simulink model "SimulinkAnalysisofCheetahTail"  (R2022a)
settings: Solver=ode4  StartTime=0.0  StopTime=1.5  FixedStep=0.001  RelTol=1e-3
undefined symbols (not defined in the file): B_cg_H, B_con_H, B_con_L, bar_len, cd_table, Cf, cl_table, g, gear_ratio, int_point_bar, int_point_tail, ITail, M_add, M_cg_H, M_cg_L, M_cg_W, Mb, Mm, Mt, psi3, rho, T_cg_H, T_fur_gap, T_length, T_width_major, T_width_minor, th2_initial, torque_constant, uncertainty_Forces, uncertainty_Position, Vf, windspeed
(part 18 of 21)

== matlab function SimulinkAnalysisofCheetahTail/Model/Forces/CD_CL_tail_3/aoa_tail_3 ==
  data: int_point_tail input; q input; dq input; aoa_tail_3 output; psi3 parameter; windspeed parameter; B_con_H parameter; B_con_L parameter; M_cg_H parameter; M_cg_L parameter; M_cg_W parameter; T_fur_gap parameter; T_length parameter; bar_len parameter
function aoa_tail_3  = aoa_tail_3( int_point_tail,q,dq, psi3, windspeed, B_con_H, B_con_L, M_cg_H, M_cg_L, M_cg_W, T_fur_gap, T_length, bar_len)
%#codegen
[x,y,z,phi1,th1,psi1,phi2,th2] = deal(q(1),q(2),q(3),q(4),q(5),q(6),q(7),q(8));
[dx,dy,dz,dphi1,dth1,dpsi1,dphi2,dth2] = deal(dq(1),dq(2),dq(3),dq(4),dq(5),dq(6),dq(7),dq(8));
%    This function was generated by the Symbolic Math Toolbox version 9.0.
%    09-Feb-2022 11:07:29

t2 = cos(phi1);
t3 = cos(phi2);
t4 = cos(psi1);
t5 = cos(psi3);
t6 = cos(th1);
t7 = cos(th2);
t8 = sin(phi1);
t9 = sin(phi2);
t10 = sin(psi1);
t11 = sin(psi3);
t12 = sin(th1);
t13 = sin(th2);
t14 = M_cg_L+x;
t15 = M_cg_W+y;
t16 = M_cg_H+z;
t24 = T_length./2.0;
t25 = bar_len./2.0;
t26 = int_point_tail./2.0;
t17 = B_con_L.*t6;
t18 = B_con_L.*t12;
t19 = t2.*t4;
t20 = t2.*t10;
t21 = t4.*t8;
t22 = t7.*t12;
t23 = t8.*t10;
t27 = B_con_H.*t2.*t6;
t29 = t6.*t14;
t30 = B_con_H.*t2.*t12;
t31 = B_con_H.*t6.*t8;
t34 = t12.*t14;
t36 = -t26;
t37 = t3.*t12.*t13;
t38 = t8.*t9.*t12;
t40 = t9.*t12.*t13;
t41 = t4.*t6.*t7;
t42 = t2.*t6.*t9;
t43 = t3.*t6.*t8;
t45 = t2.*t6.*t13;
t46 = t3.*t6.*t13;
t48 = t6.*t7.*t10;
t49 = t6.*t8.*t9;
t54 = t2.*t6.*t15;
t56 = t2.*t6.*t16;
t59 = t6.*t8.*t15;
t60 = t2.*t12.*t16;
t61 = t6.*t8.*t16;
t63 = t8.*t12.*t15;
t69 = t2.*t3.*t6.*t7;
t80 = t4.*t6.*t9.*t13;
t83 = t6.*t9.*t10.*t13;
t28 = t4.*t17;
t32 = t4.*t18;
t33 = t10.*t17;
t35 = t10.*t18;
t39 = t12.*t23;
t44 = t12.*t19;
t47 = t3.*t22;
t50 = t12.*t20;
t51 = t12.*t21;
t52 = B_con_H.*t6.*t19;
t53 = t4.*t29;
t55 = B_con_H.*t6.*t20;
t57 = t4.*t34;
t58 = t10.*t29;
t62 = t10.*t34;
t64 = -t30;
t65 = -t31;
t66 = -t38;
t68 = -t40;
t70 = t3.*t41;
t71 = t3.*t45;
t73 = t7.*t42;
t74 = t7.*t43;
t75 = t4.*t46;
t76 = t3.*t48;
t77 = t6.*t9.*t21;
t78 = t4.*t37;
t79 = t10.*t46;
t81 = t6.*t9.*t23;
t82 = t10.*t37;
t85 = -t48;
t86 = t6.*t16.*t19;
t87 = t6.*t15.*t21;
t88 = t6.*t16.*t20;
t89 = t6.*t15.*t23;
t90 = -t54;
t91 = -t59;
t92 = -t60;
t93 = -t61;
t94 = t3.*t6.*t7.*t19;
t95 = t3.*t6.*t7.*t20;
t96 = -t69;
t101 = t22+t45;
t120 = t24+t25+t36;
t67 = -t39;
t72 = t2.*t47;
t84 = -t44;
t97 = -t75;
t98 = -t76;
t99 = -t87;
t100 = -t89;
t102 = t20+t51;
t103 = t21+t50;
t104 = -t94;
t105 = -t95;
t111 = t11.*t101;
t115 = t42+t74;
t119 = t47+t71;
t155 = t37+t49+t96;
t157 = t43+t68+t73;
t106 = B_con_H.*t102;
t107 = B_con_H.*t103;
t108 = t19+t67;
t109 = t23+t84;
t110 = t3.*t102;
t112 = t9.*t102;
t113 = t9.*t103;
t114 = t13.*t103;
t121 = t15.*t102;
t122 = t15.*t103;
t123 = t16.*t102;
t124 = t16.*t103;
t126 = t3.*t7.*t103;
t130 = -t111;
t134 = T_fur_gap.*t115;
t135 = T_fur_gap.*t119;
t136 = int_point_tail.*t115;
t137 = int_point_tail.*t119;
t156 = t46+t66+t72;
t159 = T_fur_gap.*t155;
t161 = T_fur_gap.*t157;
t162 = int_point_tail.*t155;
t164 = int_point_tail.*t157;
t167 = t5.*t157;
t174 = t77+t78+t104;
t175 = t81+t82+t105;
t180 = t115.*t120;
t181 = t119.*t120;
t188 = t120.*t155;
t190 = t120.*t157;
t116 = B_con_H.*t108;
t117 = B_con_H.*t109;
t118 = -t107;
t125 = t7.*t110;
t127 = t3.*t114;
t128 = t7.*t113;
t129 = t3.*t108;
t131 = t9.*t108;
t132 = t9.*t109;
t133 = t13.*t109;
t138 = t15.*t108;
t139 = t15.*t109;
t140 = -t122;
t141 = t16.*t108;
t142 = t16.*t109;
t143 = -t124;
t145 = t3.*t7.*t109;
t154 = t85+t114;
t160 = T_fur_gap.*t156;
t163 = int_point_tail.*t156;
t166 = -t11.*(t48-t114);
t176 = T_fur_gap.*t174;
t177 = int_point_tail.*t174;
t178 = T_fur_gap.*t175;
t179 = int_point_tail.*t175;
t189 = t120.*t156;
t195 = t130+t167;
t206 = t120.*t174;
t207 = t120.*t175;
t220 = t135+t137+t181;
t223 = t161+t164+t190;
t224 = t65+t90+t93+t134+t136+t180;
t227 = t18+t27+t34+t56+t91+t159+t162+t188;
t144 = t7.*t129;
t146 = -t125;
t147 = t3.*t133;
t148 = t7.*t132;
t149 = -t129;
t150 = -t138;
t151 = -t139;
t158 = t41+t133;
t169 = t98+t127;
t171 = -T_fur_gap.*(t76-t127);
t173 = -int_point_tail.*(t76-t127);
t185 = -T_fur_gap.*(t125-t132);
t187 = -int_point_tail.*(t125-t132);
t191 = t79+t126+t131;
t194 = t97+t112+t145;
t199 = -t120.*(t76-t127);
t214 = -t120.*(t125-t132);
t228 = t17+t29+t63+t64+t92+t160+t163+t189;
t229 = t35+t55+t62+t88+t100+t178+t179+t207;
t230 = t32+t52+t57+t86+t99+t176+t177+t206;
t152 = -t144;
t153 = -t148;
t165 = t11.*t158;
t168 = t70+t147;
t183 = t132+t146;
t192 = T_fur_gap.*t191;
t193 = int_point_tail.*t191;
t197 = t83+t128+t149;
t200 = T_fur_gap.*t194;
t202 = int_point_tail.*t194;
t215 = t120.*t191;
t216 = t120.*t194;
t226 = t171+t173+t199;
t233 = t106+t123+t151+t185+t187+t214;
t170 = T_fur_gap.*t168;
t172 = int_point_tail.*t168;
t182 = t113+t152;
t196 = t80+t110+t153;
t198 = t120.*t168;
t203 = T_fur_gap.*t197;
t205 = int_point_tail.*t197;
t209 = t5.*t197;
t210 = -t200;
t211 = -t202;
t218 = t120.*t197;
t219 = -t216;
t235 = t33+t58+t118+t143+t150+t192+t193+t215;
t184 = T_fur_gap.*t182;
t186 = int_point_tail.*t182;
t201 = T_fur_gap.*t196;
t204 = int_point_tail.*t196;
t208 = t5.*t196;
t212 = -t209;
t213 = t120.*t182;
t217 = t120.*t196;
t225 = t170+t172+t198;
t232 = t203+t205+t218;
t236 = t28+t53+t117+t121+t142+t210+t211+t219;
t221 = t165+t208;
t222 = t166+t212;
t231 = t201+t204+t217;
t234 = t116+t140+t141+t184+t186+t213;
et1 = dphi1.*(t234.*(t209+t11.*(t48-t114))+(t111-t167).*(t31+t54+t61-t134-t136-t180)+t221.*(-t106-t123+t139+T_fur_gap.*(t125-t132)+int_point_tail.*(t125-t132)+t120.*(t125-t132))-t227.*(t5.*(t7.*t49-t2.*t3.*t6)-t6.*t8.*t11.*t13)+t236.*(t5.*(t3.*t109+t7.*t112)-t11.*t13.*t102)-t235.*(t5.*(t3.*t103+t7.*t131)-t11.*t13.*t108))+dphi2.*(t232.*(t209+t11.*(t48-t114))+t221.*t231-t223.*(t111-t167)-t5.*t155.*t227-t5.*t191.*t235+t5.*t194.*t236);
et2 = dth1.*(t229.*(t209+t11.*(t48-t114))+t221.*t230-t228.*(t111-t167)-t227.*(t11.*(t6.*t7-t2.*t12.*t13)+t5.*(t3.*t8.*t12+t6.*t9.*t13+t2.*t9.*t22))+t236.*(t11.*(t4.*t22+t6.*t13.*t19)-t5.*(t4.*t68+t3.*t6.*t21+t6.*t7.*t9.*t19))+t235.*(t11.*(t10.*t22+t6.*t13.*t20)-t5.*(t10.*t68+t3.*t6.*t23+t6.*t7.*t9.*t20)))+dy.*(t108.*(t209+t11.*(t48-t114))-t102.*t221+t6.*t8.*(t111-t167))-dz.*(-t103.*(t209+t11.*(t48-t114))+t109.*t221+t2.*t6.*(t111-t167));
et3 = -dth2.*(-t227.*(t11.*(t12.*t13-t2.*t6.*t7)-t5.*(t9.*t22+t13.*t42))-t235.*(t11.*(t7.*t103+t6.*t10.*t13)-t5.*(t9.*t48-t13.*t113))+t236.*(t11.*(t7.*t109-t4.*t6.*t13)+t5.*(t9.*t41+t13.*t132))+t221.*t225+(t209+t11.*(t48-t114)).*(T_fur_gap.*(t76-t127)+int_point_tail.*(t76-t127)+t120.*(t76-t127))+t220.*(t111-t167))-dx.*(t12.*(t111-t167)+t6.*t10.*(t209+t11.*(t48-t114))+t4.*t6.*t221)+t5.*windspeed.*(t209+t11.*(t48-t114))+t11.*t221.*windspeed;
et4 = -dphi1.*(t155.*(t31+t54+t61-t134-t136-t180)-t115.*t227+t182.*t235+t191.*t234+t236.*(t125-t132)-t194.*(-t106-t123+t139+T_fur_gap.*(t125-t132)+int_point_tail.*(t125-t132)+t120.*(t125-t132)))+dth2.*(t119.*t227+t155.*t220+t168.*t236-t194.*t225+t191.*(T_fur_gap.*(t76-t127)+int_point_tail.*(t76-t127)+t120.*(t76-t127))+t235.*(t76-t127))-dy.*(t102.*t194+t108.*t191+t6.*t8.*t155)-dz.*(t103.*t191+t109.*t194-t2.*t6.*t155)+dphi2.*(t155.*t223+t157.*t227-t191.*t232+t194.*t231-t196.*t236-t197.*t235);
et5 = dth1.*(t155.*t228+t156.*t227-t174.*t236-t175.*t235-t191.*t229+t194.*t230)+dx.*(t12.*t155-t4.*t6.*t194+t6.*t10.*t191)-t5.*t191.*windspeed+t11.*t194.*windspeed;
aoa_tail_3 = th2-atan((et4+et5)./(et1+et2+et3));

== matlab function SimulinkAnalysisofCheetahTail/Model/Forces/CD_CL_tail_4/v_tail_4 ==
  data: int_point_tail input; q input; dq input; v_tail_4_speed output; psi3 parameter; windspeed parameter; B_con_H parameter; B_con_L parameter; M_cg_H parameter; M_cg_L parameter; M_cg_W parameter; T_fur_gap parameter; T_length parameter; bar_len parameter
function v_tail_4_speed = v_tail_4(int_point_tail,q,dq, psi3, windspeed, B_con_H, B_con_L, M_cg_H, M_cg_L, M_cg_W, T_fur_gap, T_length, bar_len)
%#codegen
[x,y,z,phi1,th1,psi1,phi2,th2] = deal(q(1),q(2),q(3),q(4),q(5),q(6),q(7),q(8));
[dx,dy,dz,dphi1,dth1,dpsi1,dphi2,dth2] = deal(dq(1),dq(2),dq(3),dq(4),dq(5),dq(6),dq(7),dq(8));
%    This function was generated by the Symbolic Math Toolbox version 9.0.
%    09-Feb-2022 11:07:32

t2 = cos(phi1);
t3 = cos(phi2);
t4 = cos(psi1);
t5 = cos(psi3);
t6 = cos(th1);
t7 = cos(th2);
t8 = sin(phi1);
t9 = sin(phi2);
t10 = sin(psi1);
t11 = sin(psi3);
t12 = sin(th1);
t13 = sin(th2);
t14 = M_cg_L+x;
t15 = M_cg_W+y;
t16 = M_cg_H+z;
t35 = T_length.*(7.0./1.0e+1);
t36 = bar_len.*(7.0./1.0e+1);
t37 = int_point_tail.*(7.0./1.0e+1);
t17 = B_con_L.*t6;
t18 = B_con_L.*t12;
t19 = t2.*t4;
t20 = t6.*t7;
t21 = t2.*t10;
t22 = t4.*t8;
t23 = t7.*t12;
t24 = t8.*t10;
t25 = t12.*t13;
t26 = B_con_H.*t2.*t6;
t28 = t6.*t14;
t29 = B_con_H.*t2.*t12;
t30 = B_con_H.*t6.*t8;
t33 = t12.*t14;
t40 = t6.*t9.*t13;
t42 = t6.*t10.*t13;
t44 = t8.*t9.*t12;
t47 = -t37;
t48 = t2.*t3.*t6;
t51 = t2.*t6.*t9;
t52 = t3.*t6.*t8;
t54 = t2.*t6.*t13;
t55 = t3.*t6.*t13;
t57 = t4.*t6.*t13;
t60 = t3.*t8.*t12;
t61 = t6.*t8.*t9;
t66 = t2.*t6.*t15;
t68 = t2.*t6.*t16;
t71 = t6.*t8.*t15;
t72 = t2.*t12.*t16;
t73 = t6.*t8.*t16;
t75 = t8.*t12.*t15;
t27 = t4.*t17;
t31 = t4.*t18;
t32 = t10.*t17;
t34 = t10.*t18;
t38 = t2.*t25;
t39 = t3.*t25;
t41 = t9.*t23;
t43 = t10.*t23;
t45 = t12.*t24;
t46 = t9.*t25;
t49 = t2.*t20;
t50 = t4.*t20;
t53 = t12.*t19;
t56 = t3.*t23;
t58 = t4.*t23;
t59 = t10.*t20;
t62 = t12.*t21;
t63 = t12.*t22;
t64 = B_con_H.*t6.*t19;
t65 = t4.*t28;
t67 = B_con_H.*t6.*t21;
t69 = t4.*t33;
t70 = t10.*t28;
t74 = t10.*t33;
t76 = -t29;
t77 = -t30;
t79 = -t44;
t84 = t3.*t6.*t22;
t85 = t13.*t48;
t88 = t3.*t8.*t20;
t89 = t6.*t13.*t19;
t90 = t4.*t55;
t93 = t3.*t6.*t24;
t94 = t6.*t9.*t22;
t95 = t2.*t40;
t97 = t8.*t9.*t20;
t98 = t6.*t13.*t21;
t100 = t3.*t42;
t101 = t4.*t40;
t103 = t6.*t9.*t24;
t107 = t10.*t40;
t109 = -t57;
t112 = t6.*t16.*t19;
t113 = t6.*t15.*t22;
t114 = t6.*t16.*t21;
t115 = t6.*t15.*t24;
t116 = -t66;
t117 = -t71;
t118 = -t72;
t119 = -t73;
t120 = t3.*t19.*t20;
t121 = t3.*t20.*t21;
t122 = t9.*t19.*t20;
t123 = t9.*t20.*t21;
t133 = t23+t54;
t194 = t35+t36+t47;
t78 = -t38;
t80 = -t45;
t81 = -t46;
t82 = t3.*t49;
t83 = t3.*t50;
t86 = t2.*t56;
t87 = t9.*t49;
t91 = t3.*t59;
t92 = t9.*t50;
t96 = t2.*t41;
t99 = t4.*t39;
t102 = t9.*t59;
t104 = -t49;
t105 = t10.*t39;
t106 = t4.*t46;
t108 = -t53;
t110 = -t59;
t111 = t10.*t46;
t125 = -t90;
t127 = -t97;
t131 = -t113;
t132 = -t115;
t134 = t21+t63;
t135 = t22+t62;
t136 = -t120;
t137 = -t121;
t144 = t5.*t133;
t148 = t11.*t133;
t152 = t51+t88;
t156 = t56+t85;
t157 = t58+t89;
t158 = t41+t95;
t159 = t43+t98;
t124 = -t82;
t126 = -t91;
t128 = -t102;
t129 = t4.*t81;
t130 = t10.*t81;
t138 = B_con_H.*t134;
t139 = B_con_H.*t135;
t140 = t20+t78;
t141 = t25+t104;
t142 = t19+t80;
t143 = t24+t108;
t145 = t3.*t134;
t146 = t3.*t135;
t147 = t7.*t135;
t149 = t9.*t134;
t150 = t9.*t135;
t151 = t13.*t135;
t160 = t15.*t134;
t161 = t15.*t135;
t162 = t16.*t134;
t163 = t16.*t135;
t173 = -t148;
t177 = t48+t127;
t178 = T_fur_gap.*t152;
t179 = T_fur_gap.*t156;
t180 = int_point_tail.*t152;
t181 = int_point_tail.*t156;
t202 = t40+t60+t96;
t205 = t55+t79+t86;
t206 = t52+t81+t87;
t229 = t94+t99+t136;
t231 = t103+t105+t137;
t239 = t152.*t194;
t240 = t156.*t194;
t153 = B_con_H.*t142;
t154 = B_con_H.*t143;
t155 = -t139;
t164 = t7.*t145;
t165 = t7.*t146;
t166 = t13.*t146;
t167 = t7.*t149;
t168 = t9.*t147;
t169 = t13.*t150;
t170 = t3.*t142;
t171 = t3.*t143;
t172 = t7.*t143;
t174 = t9.*t142;
t175 = t9.*t143;
t176 = t13.*t143;
t182 = t15.*t142;
t183 = t15.*t143;
t184 = -t161;
t185 = t16.*t142;
t186 = t16.*t143;
t187 = -t163;
t201 = t42+t147;
t203 = t110+t151;
t204 = t39+t61+t124;
t209 = T_fur_gap.*t205;
t210 = T_fur_gap.*t206;
t212 = int_point_tail.*t205;
t213 = int_point_tail.*t206;
t216 = -t5.*(t59-t151);
t218 = -t11.*(t59-t151);
t219 = t5.*t206;
t220 = t11.*t206;
t230 = t84+t122+t129;
t232 = t93+t123+t130;
t233 = T_fur_gap.*t229;
t234 = int_point_tail.*t229;
t235 = T_fur_gap.*t231;
t236 = int_point_tail.*t231;
t250 = t194.*t205;
t251 = t194.*t206;
t272 = t194.*t229;
t275 = t194.*t231;
t283 = t179+t181+t240;
t289 = t77+t116+t119+t178+t180+t239;
t188 = t7.*t170;
t189 = t7.*t171;
t190 = -t164;
t191 = t13.*t171;
t192 = t7.*t174;
t193 = t9.*t172;
t195 = t13.*t175;
t196 = -t170;
t197 = -t182;
t198 = -t183;
t207 = t50+t176;
t208 = T_fur_gap.*t204;
t211 = int_point_tail.*t204;
t214 = t109+t172;
t222 = t126+t166;
t224 = t128+t169;
t226 = -T_fur_gap.*(t91-t166);
t228 = -int_point_tail.*(t91-t166);
t238 = t167+t171;
t244 = -T_fur_gap.*(t164-t175);
t246 = -int_point_tail.*(t164-t175);
t247 = t144+t220;
t248 = t100+t165+t174;
t249 = t194.*t204;
t255 = t173+t219;
t268 = -t194.*(t91-t166);
t277 = -t194.*(t164-t175);
t288 = t210+t213+t251;
t293 = t17+t28+t75+t76+t118+t209+t212+t250;
t294 = t34+t67+t74+t114+t132+t235+t236+t275;
t295 = t31+t64+t69+t112+t131+t233+t234+t272;
t199 = -t188;
t200 = -t193;
t215 = t5.*t207;
t217 = t11.*t207;
t221 = t83+t191;
t223 = t92+t195;
t237 = t146+t192;
t242 = t175+t190;
t252 = T_fur_gap.*t248;
t253 = int_point_tail.*t248;
t254 = t125+t149+t189;
t257 = t107+t168+t196;
t278 = t194.*t248;
t291 = t226+t228+t268;
t292 = t18+t26+t33+t68+t117+t208+t211+t249;
t298 = t138+t162+t198+t244+t246+t277;
t225 = T_fur_gap.*t221;
t227 = int_point_tail.*t221;
t241 = t150+t199;
t256 = t101+t145+t200;
t258 = T_fur_gap.*t254;
t260 = int_point_tail.*t254;
t261 = T_fur_gap.*t257;
t263 = int_point_tail.*t257;
t265 = t194.*t221;
t266 = t5.*t257;
t269 = t11.*t257;
t279 = t194.*t254;
t281 = t194.*t257;
t300 = t32+t70+t155+t187+t197+t252+t253+t278;
t243 = T_fur_gap.*t241;
t245 = int_point_tail.*t241;
t259 = T_fur_gap.*t256;
t262 = int_point_tail.*t256;
t264 = t5.*t256;
t267 = t11.*t256;
t270 = -t258;
t271 = -t260;
t273 = -t266;
t276 = t194.*t241;
t280 = t194.*t256;
t282 = -t279;
t285 = t216+t269;
t290 = t225+t227+t265;
t297 = t261+t263+t281;
t274 = -t267;
t284 = t217+t264;
t287 = t218+t273;
t296 = t259+t262+t280;
t299 = t153+t184+t185+t243+t245+t276;
t301 = t27+t65+t154+t160+t186+t270+t271+t282;
t286 = t215+t274;
et1 = dphi1.*(t204.*(t30+t66+t73-t178-t180-t239)-t152.*t292+t241.*t300+t248.*t299+t301.*(t164-t175)-t254.*(-t138-t162+t183+T_fur_gap.*(t164-t175)+int_point_tail.*(t164-t175)+t194.*(t164-t175)))-dth2.*(t156.*t292+t204.*t283+t221.*t301-t254.*t290+t248.*(T_fur_gap.*(t91-t166)+int_point_tail.*(t91-t166)+t194.*(t91-t166))+t300.*(t91-t166))+dy.*(t134.*t254+t142.*t248+t6.*t8.*t204)+dz.*(t135.*t248+t143.*t254-t2.*t6.*t204)-dphi2.*(t204.*t288+t206.*t292-t248.*t297+t254.*t296-t256.*t301-t257.*t300);
et2 = -dth1.*(t204.*t293+t205.*t292-t229.*t301-t231.*t300-t248.*t294+t254.*t295)-dx.*(t12.*t204-t4.*t6.*t254+t6.*t10.*t248)+t5.*t248.*windspeed-t11.*t254.*windspeed;
et3 = dphi2.*(t297.*(t269-t5.*(t59-t151))+t247.*t288-t286.*t296-t11.*t204.*t292-t11.*t248.*t300+t11.*t254.*t301)+dth1.*(t294.*(t269-t5.*(t59-t151))+t247.*t293-t286.*t295+t292.*(t5.*t140-t11.*t202)-t301.*(t5.*t157+t11.*t230)-t300.*(t5.*t159+t11.*t232))+dy.*(t142.*(t269-t5.*(t59-t151))+t134.*t286-t6.*t8.*t247)+dz.*(t135.*(t269-t5.*(t59-t151))+t143.*t286+t2.*t6.*t247);
et4 = -dth2.*(-t247.*t283-t286.*t290+(t269-t5.*(t59-t151)).*(T_fur_gap.*(t91-t166)+int_point_tail.*(t91-t166)+t194.*(t91-t166))+t292.*(t5.*t141+t11.*t158)+t301.*(t11.*t223+t5.*(t57-t172))+t300.*(t5.*t201+t11.*(t102-t169)))+dx.*(t12.*t247-t6.*t10.*(t269-t5.*(t59-t151))+t4.*t6.*t286);
et5 = -dphi1.*(t247.*(t30+t66+t73-t178-t180-t239)-t299.*(t269-t5.*(t59-t151))-t301.*(t11.*t238+t5.*t13.*t134)+t300.*(t11.*t237+t5.*t13.*t142)+t286.*(-t138-t162+t183+T_fur_gap.*(t164-t175)+int_point_tail.*(t164-t175)+t194.*(t164-t175))-t292.*(t11.*t177-t5.*t6.*t8.*t13))+t5.*windspeed.*(t269-t5.*(t59-t151))-t11.*t286.*windspeed;
et6 = -dphi1.*(t299.*(t266+t11.*(t59-t151))+t301.*(t5.*t238-t11.*t13.*t134)-t300.*(t5.*t237-t11.*t13.*t142)+(t148-t219).*(t30+t66+t73-t178-t180-t239)+t284.*(-t138-t162+t183+T_fur_gap.*(t164-t175)+int_point_tail.*(t164-t175)+t194.*(t164-t175))+t292.*(t5.*t177+t6.*t8.*t11.*t13))-dphi2.*(t297.*(t266+t11.*(t59-t151))+t284.*t296-t288.*(t148-t219)-t5.*t204.*t292-t5.*t248.*t300+t5.*t254.*t301);
et7 = -dth1.*(t294.*(t266+t11.*(t59-t151))+t284.*t295-t293.*(t148-t219)-t292.*(t11.*t140+t5.*t202)+t301.*(t11.*t157-t5.*t230)+t300.*(t11.*t159-t5.*t232))-dy.*(t142.*(t266+t11.*(t59-t151))-t134.*t284+t6.*t8.*(t148-t219))+dz.*(-t135.*(t266+t11.*(t59-t151))+t143.*t284+t2.*t6.*(t148-t219));
et8 = dth2.*(t284.*t290+(t266+t11.*(t59-t151)).*(T_fur_gap.*(t91-t166)+int_point_tail.*(t91-t166)+t194.*(t91-t166))+t283.*(t148-t219)-t292.*(t11.*t141-t5.*t158)+t301.*(t5.*t223-t11.*(t57-t172))-t300.*(t11.*t201-t5.*(t102-t169)))+dx.*(t12.*(t148-t219)+t6.*t10.*(t266+t11.*(t59-t151))+t4.*t6.*t284)-t5.*windspeed.*(t266+t11.*(t59-t151))-t11.*t284.*windspeed;
v_tail_4_speed = sqrt(abs(et3+et4+et5).^2+abs(et6+et7+et8).^2+abs(et1+et2).^2);

== matlab function SimulinkAnalysisofCheetahTail/Model/Forces/CD_CL_tail_4/aoa_tail_4 ==
  data: int_point_tail input; q input; dq input; aoa_tail_4 output; psi3 parameter; windspeed parameter; B_con_H parameter; B_con_L parameter; M_cg_H parameter; M_cg_L parameter; M_cg_W parameter; T_fur_gap parameter; T_length parameter; bar_len parameter
function aoa_tail_4 = aoa_tail_4(int_point_tail,q,dq, psi3, windspeed, B_con_H, B_con_L, M_cg_H, M_cg_L, M_cg_W, T_fur_gap, T_length, bar_len)
%#codegen
[x,y,z,phi1,th1,psi1,phi2,th2] = deal(q(1),q(2),q(3),q(4),q(5),q(6),q(7),q(8));
[dx,dy,dz,dphi1,dth1,dpsi1,dphi2,dth2] = deal(dq(1),dq(2),dq(3),dq(4),dq(5),dq(6),dq(7),dq(8));
%    This function was generated by the Symbolic Math Toolbox version 9.0.
%    09-Feb-2022 11:07:35

t2 = cos(phi1);
t3 = cos(phi2);
t4 = cos(psi1);
t5 = cos(psi3);
t6 = cos(th1);
t7 = cos(th2);
t8 = sin(phi1);
t9 = sin(phi2);
t10 = sin(psi1);
t11 = sin(psi3);
t12 = sin(th1);
t13 = sin(th2);
t14 = M_cg_L+x;
t15 = M_cg_W+y;
t16 = M_cg_H+z;
t33 = T_length.*(7.0./1.0e+1);
t34 = bar_len.*(7.0./1.0e+1);
t35 = int_point_tail.*(7.0./1.0e+1);
t17 = B_con_L.*t6;
t18 = B_con_L.*t12;
t19 = t2.*t4;
t20 = t2.*t10;
t21 = t4.*t8;
t22 = t7.*t12;
t23 = t8.*t10;
t24 = B_con_H.*t2.*t6;
t26 = t6.*t14;
t27 = B_con_H.*t2.*t12;
t28 = B_con_H.*t6.*t8;
t31 = t12.*t14;
t36 = t3.*t12.*t13;
t37 = t8.*t9.*t12;
t39 = t9.*t12.*t13;
t40 = -t35;
t41 = t4.*t6.*t7;
t42 = t2.*t6.*t9;
t43 = t3.*t6.*t8;
t45 = t2.*t6.*t13;
t46 = t3.*t6.*t13;
t48 = t6.*t7.*t10;
t49 = t6.*t8.*t9;
t54 = t2.*t6.*t15;
t56 = t2.*t6.*t16;
t59 = t6.*t8.*t15;
t60 = t2.*t12.*t16;
t61 = t6.*t8.*t16;
t63 = t8.*t12.*t15;
t69 = t2.*t3.*t6.*t7;
t80 = t4.*t6.*t9.*t13;
t83 = t6.*t9.*t10.*t13;
t25 = t4.*t17;
t29 = t4.*t18;
t30 = t10.*t17;
t32 = t10.*t18;
t38 = t12.*t23;
t44 = t12.*t19;
t47 = t3.*t22;
t50 = t12.*t20;
t51 = t12.*t21;
t52 = B_con_H.*t6.*t19;
t53 = t4.*t26;
t55 = B_con_H.*t6.*t20;
t57 = t4.*t31;
t58 = t10.*t26;
t62 = t10.*t31;
t64 = -t27;
t65 = -t28;
t66 = -t37;
t68 = -t39;
t70 = t3.*t41;
t71 = t3.*t45;
t73 = t7.*t42;
t74 = t7.*t43;
t75 = t4.*t46;
t76 = t3.*t48;
t77 = t6.*t9.*t21;
t78 = t4.*t36;
t79 = t10.*t46;
t81 = t6.*t9.*t23;
t82 = t10.*t36;
t85 = -t48;
t86 = t6.*t16.*t19;
t87 = t6.*t15.*t21;
t88 = t6.*t16.*t20;
t89 = t6.*t15.*t23;
t90 = -t54;
t91 = -t59;
t92 = -t60;
t93 = -t61;
t94 = t3.*t6.*t7.*t19;
t95 = t3.*t6.*t7.*t20;
t96 = -t69;
t101 = t22+t45;
t148 = t33+t34+t40;
t67 = -t38;
t72 = t2.*t47;
t84 = -t44;
t97 = -t75;
t98 = -t76;
t99 = -t87;
t100 = -t89;
t102 = t20+t51;
t103 = t21+t50;
t104 = -t94;
t105 = -t95;
t111 = t11.*t101;
t115 = t42+t74;
t119 = t47+t71;
t155 = t36+t49+t96;
t157 = t43+t68+t73;
t106 = B_con_H.*t102;
t107 = B_con_H.*t103;
t108 = t19+t67;
t109 = t23+t84;
t110 = t3.*t102;
t112 = t9.*t102;
t113 = t9.*t103;
t114 = t13.*t103;
t120 = t15.*t102;
t121 = t15.*t103;
t122 = t16.*t102;
t123 = t16.*t103;
t125 = t3.*t7.*t103;
t129 = -t111;
t133 = T_fur_gap.*t115;
t134 = T_fur_gap.*t119;
t135 = int_point_tail.*t115;
t136 = int_point_tail.*t119;
t156 = t46+t66+t72;
t159 = T_fur_gap.*t155;
t161 = T_fur_gap.*t157;
t162 = int_point_tail.*t155;
t164 = int_point_tail.*t157;
t167 = t5.*t157;
t174 = t77+t78+t104;
t175 = t81+t82+t105;
t180 = t115.*t148;
t181 = t119.*t148;
t189 = t148.*t155;
t191 = t148.*t157;
t116 = B_con_H.*t108;
t117 = B_con_H.*t109;
t118 = -t107;
t124 = t7.*t110;
t126 = t3.*t114;
t127 = t7.*t113;
t128 = t3.*t108;
t130 = t9.*t108;
t131 = t9.*t109;
t132 = t13.*t109;
t137 = t15.*t108;
t138 = t15.*t109;
t139 = -t121;
t140 = t16.*t108;
t141 = t16.*t109;
t142 = -t123;
t144 = t3.*t7.*t109;
t154 = t85+t114;
t160 = T_fur_gap.*t156;
t163 = int_point_tail.*t156;
t166 = -t11.*(t48-t114);
t176 = T_fur_gap.*t174;
t177 = int_point_tail.*t174;
t178 = T_fur_gap.*t175;
t179 = int_point_tail.*t175;
t190 = t148.*t156;
t195 = t129+t167;
t210 = t148.*t174;
t212 = t148.*t175;
t220 = t134+t136+t181;
t223 = t161+t164+t191;
t224 = t65+t90+t93+t133+t135+t180;
t227 = t18+t24+t31+t56+t91+t159+t162+t189;
t143 = t7.*t128;
t145 = -t124;
t146 = t3.*t132;
t147 = t7.*t131;
t149 = -t128;
t150 = -t137;
t151 = -t138;
t158 = t41+t132;
t169 = t98+t126;
t171 = -T_fur_gap.*(t76-t126);
t173 = -int_point_tail.*(t76-t126);
t185 = -T_fur_gap.*(t124-t131);
t187 = -int_point_tail.*(t124-t131);
t188 = t79+t125+t130;
t194 = t97+t112+t144;
t207 = -t148.*(t76-t126);
t214 = -t148.*(t124-t131);
t228 = t17+t26+t63+t64+t92+t160+t163+t190;
t229 = t32+t55+t62+t88+t100+t178+t179+t212;
t230 = t29+t52+t57+t86+t99+t176+t177+t210;
t152 = -t143;
t153 = -t147;
t165 = t11.*t158;
t168 = t70+t146;
t183 = t131+t145;
t192 = T_fur_gap.*t188;
t193 = int_point_tail.*t188;
t197 = t83+t127+t149;
t198 = T_fur_gap.*t194;
t200 = int_point_tail.*t194;
t215 = t148.*t188;
t216 = t148.*t194;
t226 = t171+t173+t207;
t233 = t106+t122+t151+t185+t187+t214;
t170 = T_fur_gap.*t168;
t172 = int_point_tail.*t168;
t182 = t113+t152;
t196 = t80+t110+t153;
t201 = T_fur_gap.*t197;
t203 = int_point_tail.*t197;
t205 = t148.*t168;
t206 = t5.*t197;
t208 = -t198;
t209 = -t200;
t218 = t148.*t197;
t219 = -t216;
t235 = t30+t58+t118+t142+t150+t192+t193+t215;
t184 = T_fur_gap.*t182;
t186 = int_point_tail.*t182;
t199 = T_fur_gap.*t196;
t202 = int_point_tail.*t196;
t204 = t5.*t196;
t211 = -t206;
t213 = t148.*t182;
t217 = t148.*t196;
t225 = t170+t172+t205;
t232 = t201+t203+t218;
t236 = t25+t53+t117+t120+t141+t208+t209+t219;
t221 = t165+t204;
t222 = t166+t211;
t231 = t199+t202+t217;
t234 = t116+t139+t140+t184+t186+t213;
et1 = dphi1.*(t234.*(t206+t11.*(t48-t114))+(t111-t167).*(t28+t54+t61-t133-t135-t180)+t221.*(-t106-t122+t138+T_fur_gap.*(t124-t131)+int_point_tail.*(t124-t131)+t148.*(t124-t131))-t227.*(t5.*(t7.*t49-t2.*t3.*t6)-t6.*t8.*t11.*t13)+t236.*(t5.*(t3.*t109+t7.*t112)-t11.*t13.*t102)-t235.*(t5.*(t3.*t103+t7.*t130)-t11.*t13.*t108))+dphi2.*(t232.*(t206+t11.*(t48-t114))+t221.*t231-t223.*(t111-t167)-t5.*t155.*t227-t5.*t188.*t235+t5.*t194.*t236);
et2 = dth1.*(t229.*(t206+t11.*(t48-t114))+t221.*t230-t228.*(t111-t167)-t227.*(t11.*(t6.*t7-t2.*t12.*t13)+t5.*(t3.*t8.*t12+t6.*t9.*t13+t2.*t9.*t22))+t236.*(t11.*(t4.*t22+t6.*t13.*t19)-t5.*(t4.*t68+t3.*t6.*t21+t6.*t7.*t9.*t19))+t235.*(t11.*(t10.*t22+t6.*t13.*t20)-t5.*(t10.*t68+t3.*t6.*t23+t6.*t7.*t9.*t20)))+dy.*(t108.*(t206+t11.*(t48-t114))-t102.*t221+t6.*t8.*(t111-t167))-dz.*(-t103.*(t206+t11.*(t48-t114))+t109.*t221+t2.*t6.*(t111-t167));
et3 = -dth2.*(-t227.*(t11.*(t12.*t13-t2.*t6.*t7)-t5.*(t9.*t22+t13.*t42))-t235.*(t11.*(t7.*t103+t6.*t10.*t13)-t5.*(t9.*t48-t13.*t113))+t236.*(t11.*(t7.*t109-t4.*t6.*t13)+t5.*(t9.*t41+t13.*t131))+t221.*t225+(t206+t11.*(t48-t114)).*(T_fur_gap.*(t76-t126)+int_point_tail.*(t76-t126)+t148.*(t76-t126))+t220.*(t111-t167))-dx.*(t12.*(t111-t167)+t6.*t10.*(t206+t11.*(t48-t114))+t4.*t6.*t221)+t5.*windspeed.*(t206+t11.*(t48-t114))+t11.*t221.*windspeed;
et4 = -dphi1.*(t155.*(t28+t54+t61-t133-t135-t180)-t115.*t227+t182.*t235+t188.*t234+t236.*(t124-t131)-t194.*(-t106-t122+t138+T_fur_gap.*(t124-t131)+int_point_tail.*(t124-t131)+t148.*(t124-t131)))+dth2.*(t119.*t227+t155.*t220+t168.*t236-t194.*t225+t188.*(T_fur_gap.*(t76-t126)+int_point_tail.*(t76-t126)+t148.*(t76-t126))+t235.*(t76-t126))-dy.*(t102.*t194+t108.*t188+t6.*t8.*t155)-dz.*(t103.*t188+t109.*t194-t2.*t6.*t155)+dphi2.*(t155.*t223+t157.*t227-t188.*t232+t194.*t231-t196.*t236-t197.*t235);
et5 = dth1.*(t155.*t228+t156.*t227-t174.*t236-t175.*t235-t188.*t229+t194.*t230)+dx.*(t12.*t155-t4.*t6.*t194+t6.*t10.*t188)-t5.*t188.*windspeed+t11.*t194.*windspeed;
aoa_tail_4 = th2-atan((et4+et5)./(et1+et2+et3));

== matlab function SimulinkAnalysisofCheetahTail/Model/Forces/CD_CL_tail_5/v_tail_5 ==
  data: int_point_tail input; q input; dq input; v_tail_5_speed output; psi3 parameter; windspeed parameter; B_con_H parameter; B_con_L parameter; M_cg_H parameter; M_cg_L parameter; M_cg_W parameter; T_fur_gap parameter; T_length parameter; bar_len parameter
function v_tail_5_speed = v_tail_5(int_point_tail,q,dq, psi3, windspeed, B_con_H, B_con_L, M_cg_H, M_cg_L, M_cg_W, T_fur_gap, T_length, bar_len)
%#codegen
[x,y,z,phi1,th1,psi1,phi2,th2] = deal(q(1),q(2),q(3),q(4),q(5),q(6),q(7),q(8));
[dx,dy,dz,dphi1,dth1,dpsi1,dphi2,dth2] = deal(dq(1),dq(2),dq(3),dq(4),dq(5),dq(6),dq(7),dq(8));
%    This function was generated by the Symbolic Math Toolbox version 9.0.
%    09-Feb-2022 11:07:38

t2 = cos(phi1);
t3 = cos(phi2);
t4 = cos(psi1);
t5 = cos(psi3);
t6 = cos(th1);
t7 = cos(th2);
t8 = sin(phi1);
t9 = sin(phi2);
t10 = sin(psi1);
t11 = sin(psi3);
t12 = sin(th1);
t13 = sin(th2);
t14 = M_cg_L+x;
t15 = M_cg_W+y;
t16 = M_cg_H+z;
t44 = T_length.*(9.0./1.0e+1);
t45 = bar_len.*(9.0./1.0e+1);
t46 = int_point_tail.*(9.0./1.0e+1);
t17 = B_con_L.*t6;
t18 = B_con_L.*t12;
t19 = t2.*t4;
t20 = t6.*t7;
t21 = t2.*t10;
t22 = t4.*t8;
t23 = t7.*t12;
t24 = t8.*t10;
t25 = t12.*t13;
t26 = B_con_H.*t2.*t6;
t28 = t6.*t14;
t29 = B_con_H.*t2.*t12;
t30 = B_con_H.*t6.*t8;
t33 = t12.*t14;
t37 = t6.*t9.*t13;
t39 = t6.*t10.*t13;
t41 = t8.*t9.*t12;
t47 = t2.*t3.*t6;
t50 = t2.*t6.*t9;
t51 = t3.*t6.*t8;
t53 = t2.*t6.*t13;
t54 = t3.*t6.*t13;
t56 = t4.*t6.*t13;
t59 = t3.*t8.*t12;
t60 = t6.*t8.*t9;
t65 = t2.*t6.*t15;
t67 = t2.*t6.*t16;
t70 = t6.*t8.*t15;
t71 = t2.*t12.*t16;
t72 = t6.*t8.*t16;
t74 = t8.*t12.*t15;
t77 = -t46;
t27 = t4.*t17;
t31 = t4.*t18;
t32 = t10.*t17;
t34 = t10.*t18;
t35 = t2.*t25;
t36 = t3.*t25;
t38 = t9.*t23;
t40 = t10.*t23;
t42 = t12.*t24;
t43 = t9.*t25;
t48 = t2.*t20;
t49 = t4.*t20;
t52 = t12.*t19;
t55 = t3.*t23;
t57 = t4.*t23;
t58 = t10.*t20;
t61 = t12.*t21;
t62 = t12.*t22;
t63 = B_con_H.*t6.*t19;
t64 = t4.*t28;
t66 = B_con_H.*t6.*t21;
t68 = t4.*t33;
t69 = t10.*t28;
t73 = t10.*t33;
t75 = -t29;
t76 = -t30;
t79 = -t41;
t84 = t3.*t6.*t22;
t85 = t13.*t47;
t88 = t3.*t8.*t20;
t89 = t6.*t13.*t19;
t90 = t4.*t54;
t93 = t3.*t6.*t24;
t94 = t6.*t9.*t22;
t95 = t2.*t37;
t97 = t8.*t9.*t20;
t98 = t6.*t13.*t21;
t100 = t3.*t39;
t101 = t4.*t37;
t103 = t6.*t9.*t24;
t107 = t10.*t37;
t109 = -t56;
t112 = t6.*t16.*t19;
t113 = t6.*t15.*t22;
t114 = t6.*t16.*t21;
t115 = t6.*t15.*t24;
t116 = -t65;
t117 = -t70;
t118 = -t71;
t119 = -t72;
t120 = t3.*t19.*t20;
t121 = t3.*t20.*t21;
t122 = t9.*t19.*t20;
t123 = t9.*t20.*t21;
t133 = t23+t53;
t200 = t44+t45+t77;
t78 = -t35;
t80 = -t42;
t81 = -t43;
t82 = t3.*t48;
t83 = t3.*t49;
t86 = t2.*t55;
t87 = t9.*t48;
t91 = t3.*t58;
t92 = t9.*t49;
t96 = t2.*t38;
t99 = t4.*t36;
t102 = t9.*t58;
t104 = -t48;
t105 = t10.*t36;
t106 = t4.*t43;
t108 = -t52;
t110 = -t58;
t111 = t10.*t43;
t125 = -t90;
t127 = -t97;
t131 = -t113;
t132 = -t115;
t134 = t21+t62;
t135 = t22+t61;
t136 = -t120;
t137 = -t121;
t144 = t5.*t133;
t148 = t11.*t133;
t152 = t50+t88;
t156 = t55+t85;
t157 = t57+t89;
t158 = t38+t95;
t159 = t40+t98;
t124 = -t82;
t126 = -t91;
t128 = -t102;
t129 = t4.*t81;
t130 = t10.*t81;
t138 = B_con_H.*t134;
t139 = B_con_H.*t135;
t140 = t20+t78;
t141 = t25+t104;
t142 = t19+t80;
t143 = t24+t108;
t145 = t3.*t134;
t146 = t3.*t135;
t147 = t7.*t135;
t149 = t9.*t134;
t150 = t9.*t135;
t151 = t13.*t135;
t160 = t15.*t134;
t161 = t15.*t135;
t162 = t16.*t134;
t163 = t16.*t135;
t173 = -t148;
t177 = t47+t127;
t178 = T_fur_gap.*t152;
t179 = T_fur_gap.*t156;
t180 = int_point_tail.*t152;
t181 = int_point_tail.*t156;
t202 = t37+t59+t96;
t205 = t54+t79+t86;
t206 = t51+t81+t87;
t229 = t94+t99+t136;
t231 = t103+t105+t137;
t241 = t152.*t200;
t242 = t156.*t200;
t153 = B_con_H.*t142;
t154 = B_con_H.*t143;
t155 = -t139;
t164 = t7.*t145;
t165 = t7.*t146;
t166 = t13.*t146;
t167 = t7.*t149;
t168 = t9.*t147;
t169 = t13.*t150;
t170 = t3.*t142;
t171 = t3.*t143;
t172 = t7.*t143;
t174 = t9.*t142;
t175 = t9.*t143;
t176 = t13.*t143;
t182 = t15.*t142;
t183 = t15.*t143;
t184 = -t161;
t185 = t16.*t142;
t186 = t16.*t143;
t187 = -t163;
t201 = t39+t147;
t203 = t110+t151;
t204 = t36+t60+t124;
t209 = T_fur_gap.*t205;
t210 = T_fur_gap.*t206;
t212 = int_point_tail.*t205;
t213 = int_point_tail.*t206;
t216 = -t5.*(t58-t151);
t218 = -t11.*(t58-t151);
t219 = t5.*t206;
t220 = t11.*t206;
t230 = t84+t122+t129;
t232 = t93+t123+t130;
t233 = T_fur_gap.*t229;
t234 = int_point_tail.*t229;
t235 = T_fur_gap.*t231;
t236 = int_point_tail.*t231;
t258 = t200.*t205;
t259 = t200.*t206;
t274 = t200.*t229;
t275 = t200.*t231;
t283 = t179+t181+t242;
t289 = t76+t116+t119+t178+t180+t241;
t188 = t7.*t170;
t189 = t7.*t171;
t190 = -t164;
t191 = t13.*t171;
t192 = t7.*t174;
t193 = t9.*t172;
t194 = t13.*t175;
t195 = -t170;
t196 = -t182;
t197 = -t183;
t207 = t49+t176;
t208 = T_fur_gap.*t204;
t211 = int_point_tail.*t204;
t214 = t109+t172;
t222 = t126+t166;
t224 = t128+t169;
t226 = -T_fur_gap.*(t91-t166);
t228 = -int_point_tail.*(t91-t166);
t238 = t167+t171;
t244 = -T_fur_gap.*(t164-t175);
t246 = -int_point_tail.*(t164-t175);
t247 = t144+t220;
t248 = t100+t165+t174;
t252 = t173+t219;
t256 = t200.*t204;
t273 = -t200.*(t91-t166);
t277 = -t200.*(t164-t175);
t288 = t210+t213+t259;
t293 = t17+t28+t74+t75+t118+t209+t212+t258;
t294 = t34+t66+t73+t114+t132+t235+t236+t275;
t295 = t31+t63+t68+t112+t131+t233+t234+t274;
t198 = -t188;
t199 = -t193;
t215 = t5.*t207;
t217 = t11.*t207;
t221 = t83+t191;
t223 = t92+t194;
t237 = t146+t192;
t240 = t175+t190;
t249 = T_fur_gap.*t248;
t250 = int_point_tail.*t248;
t251 = t125+t149+t189;
t254 = t107+t168+t195;
t278 = t200.*t248;
t291 = t226+t228+t273;
t292 = t18+t26+t33+t67+t117+t208+t211+t256;
t298 = t138+t162+t197+t244+t246+t277;
t225 = T_fur_gap.*t221;
t227 = int_point_tail.*t221;
t239 = t150+t198;
t253 = t101+t145+t199;
t255 = T_fur_gap.*t251;
t260 = int_point_tail.*t251;
t261 = T_fur_gap.*t254;
t263 = int_point_tail.*t254;
t265 = t5.*t254;
t267 = t11.*t254;
t272 = t200.*t221;
t279 = t200.*t251;
t281 = t200.*t254;
t300 = t32+t69+t155+t187+t196+t249+t250+t278;
t243 = T_fur_gap.*t239;
t245 = int_point_tail.*t239;
t257 = T_fur_gap.*t253;
t262 = int_point_tail.*t253;
t264 = t5.*t253;
t266 = t11.*t253;
t268 = -t255;
t269 = -t260;
t270 = -t265;
t276 = t200.*t239;
t280 = t200.*t253;
t282 = -t279;
t285 = t216+t267;
t290 = t225+t227+t272;
t297 = t261+t263+t281;
t271 = -t266;
t284 = t217+t264;
t287 = t218+t270;
t296 = t257+t262+t280;
t299 = t153+t184+t185+t243+t245+t276;
t301 = t27+t64+t154+t160+t186+t268+t269+t282;
t286 = t215+t271;
et1 = dphi1.*(t204.*(t30+t65+t72-t178-t180-t241)-t152.*t292+t239.*t300+t248.*t299+t301.*(t164-t175)-t251.*(-t138-t162+t183+T_fur_gap.*(t164-t175)+int_point_tail.*(t164-t175)+t200.*(t164-t175)))-dth2.*(t156.*t292+t204.*t283+t221.*t301-t251.*t290+t248.*(T_fur_gap.*(t91-t166)+int_point_tail.*(t91-t166)+t200.*(t91-t166))+t300.*(t91-t166))+dy.*(t134.*t251+t142.*t248+t6.*t8.*t204)+dz.*(t135.*t248+t143.*t251-t2.*t6.*t204)-dphi2.*(t204.*t288+t206.*t292-t248.*t297+t251.*t296-t253.*t301-t254.*t300);
et2 = -dth1.*(t204.*t293+t205.*t292-t229.*t301-t231.*t300-t248.*t294+t251.*t295)-dx.*(t12.*t204-t4.*t6.*t251+t6.*t10.*t248)+t5.*t248.*windspeed-t11.*t251.*windspeed;
et3 = dphi2.*(t297.*(t267-t5.*(t58-t151))+t247.*t288-t286.*t296-t11.*t204.*t292-t11.*t248.*t300+t11.*t251.*t301)+dth1.*(t294.*(t267-t5.*(t58-t151))+t247.*t293-t286.*t295+t292.*(t5.*t140-t11.*t202)-t301.*(t5.*t157+t11.*t230)-t300.*(t5.*t159+t11.*t232))+dy.*(t142.*(t267-t5.*(t58-t151))+t134.*t286-t6.*t8.*t247)+dz.*(t135.*(t267-t5.*(t58-t151))+t143.*t286+t2.*t6.*t247);
et4 = -dth2.*(-t247.*t283-t286.*t290+(t267-t5.*(t58-t151)).*(T_fur_gap.*(t91-t166)+int_point_tail.*(t91-t166)+t200.*(t91-t166))+t292.*(t5.*t141+t11.*t158)+t301.*(t11.*t223+t5.*(t56-t172))+t300.*(t5.*t201+t11.*(t102-t169)))+dx.*(t12.*t247-t6.*t10.*(t267-t5.*(t58-t151))+t4.*t6.*t286);
et5 = -dphi1.*(t247.*(t30+t65+t72-t178-t180-t241)-t299.*(t267-t5.*(t58-t151))-t301.*(t11.*t238+t5.*t13.*t134)+t300.*(t11.*t237+t5.*t13.*t142)+t286.*(-t138-t162+t183+T_fur_gap.*(t164-t175)+int_point_tail.*(t164-t175)+t200.*(t164-t175))-t292.*(t11.*t177-t5.*t6.*t8.*t13))+t5.*windspeed.*(t267-t5.*(t58-t151))-t11.*t286.*windspeed;
et6 = -dphi1.*(t299.*(t265+t11.*(t58-t151))+t301.*(t5.*t238-t11.*t13.*t134)-t300.*(t5.*t237-t11.*t13.*t142)+(t148-t219).*(t30+t65+t72-t178-t180-t241)+t284.*(-t138-t162+t183+T_fur_gap.*(t164-t175)+int_point_tail.*(t164-t175)+t200.*(t164-t175))+t292.*(t5.*t177+t6.*t8.*t11.*t13))-dphi2.*(t297.*(t265+t11.*(t58-t151))+t284.*t296-t288.*(t148-t219)-t5.*t204.*t292-t5.*t248.*t300+t5.*t251.*t301);
et7 = -dth1.*(t294.*(t265+t11.*(t58-t151))+t284.*t295-t293.*(t148-t219)-t292.*(t11.*t140+t5.*t202)+t301.*(t11.*t157-t5.*t230)+t300.*(t11.*t159-t5.*t232))-dy.*(t142.*(t265+t11.*(t58-t151))-t134.*t284+t6.*t8.*(t148-t219))+dz.*(-t135.*(t265+t11.*(t58-t151))+t143.*t284+t2.*t6.*(t148-t219));
et8 = dth2.*(t284.*t290+(t265+t11.*(t58-t151)).*(T_fur_gap.*(t91-t166)+int_point_tail.*(t91-t166)+t200.*(t91-t166))+t283.*(t148-t219)-t292.*(t11.*t141-t5.*t158)+t301.*(t5.*t223-t11.*(t56-t172))-t300.*(t11.*t201-t5.*(t102-t169)))+dx.*(t12.*(t148-t219)+t6.*t10.*(t265+t11.*(t58-t151))+t4.*t6.*t284)-t5.*windspeed.*(t265+t11.*(t58-t151))-t11.*t284.*windspeed;
v_tail_5_speed = sqrt(abs(et3+et4+et5).^2+abs(et6+et7+et8).^2+abs(et1+et2).^2);

== matlab function SimulinkAnalysisofCheetahTail/Model/Forces/CD_CL_tail_5/aoa_tail_5 ==
  data: int_point_tail input; q input; dq input; aoa_tail_5 output; psi3 parameter; windspeed parameter; B_con_H parameter; B_con_L parameter; M_cg_H parameter; M_cg_L parameter; M_cg_W parameter; T_fur_gap parameter; T_length parameter; bar_len parameter
function aoa_tail_5 = aoa_tail_5(int_point_tail,q,dq, psi3, windspeed, B_con_H, B_con_L, M_cg_H, M_cg_L, M_cg_W, T_fur_gap, T_length, bar_len)
%#codegen
[x,y,z,phi1,th1,psi1,phi2,th2] = deal(q(1),q(2),q(3),q(4),q(5),q(6),q(7),q(8));
[dx,dy,dz,dphi1,dth1,dpsi1,dphi2,dth2] = deal(dq(1),dq(2),dq(3),dq(4),dq(5),dq(6),dq(7),dq(8));
%    This function was generated by the Symbolic Math Toolbox version 9.0.
%    09-Feb-2022 11:07:42

t2 = cos(phi1);
t3 = cos(phi2);
t4 = cos(psi1);
t5 = cos(psi3);
t6 = cos(th1);
t7 = cos(th2);
t8 = sin(phi1);
t9 = sin(phi2);
t10 = sin(psi1);
t11 = sin(psi3);
t12 = sin(th1);
t13 = sin(th2);
t14 = M_cg_L+x;
t15 = M_cg_W+y;
t16 = M_cg_H+z;
t37 = T_length.*(9.0./1.0e+1);
t38 = bar_len.*(9.0./1.0e+1);
t39 = int_point_tail.*(9.0./1.0e+1);
t17 = B_con_L.*t6;
t18 = B_con_L.*t12;
t19 = t2.*t4;
t20 = t2.*t10;
t21 = t4.*t8;
t22 = t7.*t12;
t23 = t8.*t10;
t24 = B_con_H.*t2.*t6;
t26 = t6.*t14;
t27 = B_con_H.*t2.*t12;
t28 = B_con_H.*t6.*t8;
t31 = t12.*t14;
t33 = t3.*t12.*t13;
t34 = t8.*t9.*t12;
t36 = t9.*t12.*t13;
t40 = t4.*t6.*t7;
t41 = t2.*t6.*t9;
t42 = t3.*t6.*t8;
t44 = t2.*t6.*t13;
t45 = t3.*t6.*t13;
t47 = t6.*t7.*t10;
t48 = t6.*t8.*t9;
t53 = t2.*t6.*t15;
t55 = t2.*t6.*t16;
t58 = t6.*t8.*t15;
t59 = t2.*t12.*t16;
t60 = t6.*t8.*t16;
t62 = t8.*t12.*t15;
t65 = -t39;
t69 = t2.*t3.*t6.*t7;
t80 = t4.*t6.*t9.*t13;
t83 = t6.*t9.*t10.*t13;
t25 = t4.*t17;
t29 = t4.*t18;
t30 = t10.*t17;
t32 = t10.*t18;
t35 = t12.*t23;
t43 = t12.*t19;
t46 = t3.*t22;
t49 = t12.*t20;
t50 = t12.*t21;
t51 = B_con_H.*t6.*t19;
t52 = t4.*t26;
t54 = B_con_H.*t6.*t20;
t56 = t4.*t31;
t57 = t10.*t26;
t61 = t10.*t31;
t63 = -t27;
t64 = -t28;
t66 = -t34;
t68 = -t36;
t70 = t3.*t40;
t71 = t3.*t44;
t73 = t7.*t41;
t74 = t7.*t42;
t75 = t4.*t45;
t76 = t3.*t47;
t77 = t6.*t9.*t21;
t78 = t4.*t33;
t79 = t10.*t45;
t81 = t6.*t9.*t23;
t82 = t10.*t33;
t85 = -t47;
t86 = t6.*t16.*t19;
t87 = t6.*t15.*t21;
t88 = t6.*t16.*t20;
t89 = t6.*t15.*t23;
t90 = -t53;
t91 = -t58;
t92 = -t59;
t93 = -t60;
t94 = t3.*t6.*t7.*t19;
t95 = t3.*t6.*t7.*t20;
t96 = -t69;
t101 = t22+t44;
t153 = t37+t38+t65;
t67 = -t35;
t72 = t2.*t46;
t84 = -t43;
t97 = -t75;
t98 = -t76;
t99 = -t87;
t100 = -t89;
t102 = t20+t50;
t103 = t21+t49;
t104 = -t94;
t105 = -t95;
t111 = t11.*t101;
t115 = t41+t74;
t119 = t46+t71;
t155 = t33+t48+t96;
t157 = t42+t68+t73;
t106 = B_con_H.*t102;
t107 = B_con_H.*t103;
t108 = t19+t67;
t109 = t23+t84;
t110 = t3.*t102;
t112 = t9.*t102;
t113 = t9.*t103;
t114 = t13.*t103;
t120 = t15.*t102;
t121 = t15.*t103;
t122 = t16.*t102;
t123 = t16.*t103;
t125 = t3.*t7.*t103;
t129 = -t111;
t133 = T_fur_gap.*t115;
t134 = T_fur_gap.*t119;
t135 = int_point_tail.*t115;
t136 = int_point_tail.*t119;
t156 = t45+t66+t72;
t159 = T_fur_gap.*t155;
t161 = T_fur_gap.*t157;
t162 = int_point_tail.*t155;
t164 = int_point_tail.*t157;
t167 = t5.*t157;
t174 = t77+t78+t104;
t175 = t81+t82+t105;
t182 = t115.*t153;
t183 = t119.*t153;
t196 = t153.*t155;
t199 = t153.*t157;
t116 = B_con_H.*t108;
t117 = B_con_H.*t109;
t118 = -t107;
t124 = t7.*t110;
t126 = t3.*t114;
t127 = t7.*t113;
t128 = t3.*t108;
t130 = t9.*t108;
t131 = t9.*t109;
t132 = t13.*t109;
t137 = t15.*t108;
t138 = t15.*t109;
t139 = -t121;
t140 = t16.*t108;
t141 = t16.*t109;
t142 = -t123;
t144 = t3.*t7.*t109;
t154 = t85+t114;
t160 = T_fur_gap.*t156;
t163 = int_point_tail.*t156;
t166 = -t11.*(t47-t114);
t176 = T_fur_gap.*t174;
t177 = int_point_tail.*t174;
t178 = T_fur_gap.*t175;
t179 = int_point_tail.*t175;
t192 = t129+t167;
t198 = t153.*t156;
t211 = t153.*t174;
t212 = t153.*t175;
t220 = t134+t136+t183;
t223 = t161+t164+t199;
t224 = t64+t90+t93+t133+t135+t182;
t227 = t18+t24+t31+t55+t91+t159+t162+t196;
t143 = t7.*t128;
t145 = -t124;
t146 = t3.*t132;
t147 = t7.*t131;
t148 = -t128;
t149 = -t137;
t150 = -t138;
t158 = t40+t132;
t169 = t98+t126;
t171 = -T_fur_gap.*(t76-t126);
t173 = -int_point_tail.*(t76-t126);
t185 = -T_fur_gap.*(t124-t131);
t187 = -int_point_tail.*(t124-t131);
t188 = t79+t125+t130;
t191 = t97+t112+t144;
t210 = -t153.*(t76-t126);
t214 = -t153.*(t124-t131);
t228 = t17+t26+t62+t63+t92+t160+t163+t198;
t229 = t32+t54+t61+t88+t100+t178+t179+t212;
t230 = t29+t51+t56+t86+t99+t176+t177+t211;
t151 = -t143;
t152 = -t147;
t165 = t11.*t158;
t168 = t70+t146;
t181 = t131+t145;
t189 = T_fur_gap.*t188;
t190 = int_point_tail.*t188;
t194 = t83+t127+t148;
t195 = T_fur_gap.*t191;
t200 = int_point_tail.*t191;
t215 = t153.*t188;
t216 = t153.*t191;
t226 = t171+t173+t210;
t233 = t106+t122+t150+t185+t187+t214;
t170 = T_fur_gap.*t168;
t172 = int_point_tail.*t168;
t180 = t113+t151;
t193 = t80+t110+t152;
t201 = T_fur_gap.*t194;
t203 = int_point_tail.*t194;
t205 = t5.*t194;
t206 = -t195;
t207 = -t200;
t209 = t153.*t168;
t218 = t153.*t194;
t219 = -t216;
t235 = t30+t57+t118+t142+t149+t189+t190+t215;
t184 = T_fur_gap.*t180;
t186 = int_point_tail.*t180;
t197 = T_fur_gap.*t193;
t202 = int_point_tail.*t193;
t204 = t5.*t193;
t208 = -t205;
t213 = t153.*t180;
t217 = t153.*t193;
t225 = t170+t172+t209;
t232 = t201+t203+t218;
t236 = t25+t52+t117+t120+t141+t206+t207+t219;
t221 = t165+t204;
t222 = t166+t208;
t231 = t197+t202+t217;
t234 = t116+t139+t140+t184+t186+t213;
et1 = dphi1.*(t234.*(t205+t11.*(t47-t114))+(t111-t167).*(t28+t53+t60-t133-t135-t182)+t221.*(-t106-t122+t138+T_fur_gap.*(t124-t131)+int_point_tail.*(t124-t131)+t153.*(t124-t131))-t227.*(t5.*(t7.*t48-t2.*t3.*t6)-t6.*t8.*t11.*t13)+t236.*(t5.*(t3.*t109+t7.*t112)-t11.*t13.*t102)-t235.*(t5.*(t3.*t103+t7.*t130)-t11.*t13.*t108))+dphi2.*(t232.*(t205+t11.*(t47-t114))+t221.*t231-t223.*(t111-t167)-t5.*t155.*t227-t5.*t188.*t235+t5.*t191.*t236);
et2 = dth1.*(t229.*(t205+t11.*(t47-t114))+t221.*t230-t228.*(t111-t167)-t227.*(t11.*(t6.*t7-t2.*t12.*t13)+t5.*(t3.*t8.*t12+t6.*t9.*t13+t2.*t9.*t22))+t236.*(t11.*(t4.*t22+t6.*t13.*t19)-t5.*(t4.*t68+t3.*t6.*t21+t6.*t7.*t9.*t19))+t235.*(t11.*(t10.*t22+t6.*t13.*t20)-t5.*(t10.*t68+t3.*t6.*t23+t6.*t7.*t9.*t20)))+dy.*(t108.*(t205+t11.*(t47-t114))-t102.*t221+t6.*t8.*(t111-t167))-dz.*(-t103.*(t205+t11.*(t47-t114))+t109.*t221+t2.*t6.*(t111-t167));
et3 = -dth2.*(-t227.*(t11.*(t12.*t13-t2.*t6.*t7)-t5.*(t9.*t22+t13.*t41))-t235.*(t11.*(t7.*t103+t6.*t10.*t13)-t5.*(t9.*t47-t13.*t113))+t236.*(t11.*(t7.*t109-t4.*t6.*t13)+t5.*(t9.*t40+t13.*t131))+t221.*t225+(t205+t11.*(t47-t114)).*(T_fur_gap.*(t76-t126)+int_point_tail.*(t76-t126)+t153.*(t76-t126))+t220.*(t111-t167))-dx.*(t12.*(t111-t167)+t6.*t10.*(t205+t11.*(t47-t114))+t4.*t6.*t221)+t5.*windspeed.*(t205+t11.*(t47-t114))+t11.*t221.*windspeed;
et4 = -dphi1.*(t155.*(t28+t53+t60-t133-t135-t182)-t115.*t227+t180.*t235+t188.*t234+t236.*(t124-t131)-t191.*(-t106-t122+t138+T_fur_gap.*(t124-t131)+int_point_tail.*(t124-t131)+t153.*(t124-t131)))+dth2.*(t119.*t227+t155.*t220+t168.*t236-t191.*t225+t188.*(T_fur_gap.*(t76-t126)+int_point_tail.*(t76-t126)+t153.*(t76-t126))+t235.*(t76-t126))-dy.*(t102.*t191+t108.*t188+t6.*t8.*t155)-dz.*(t103.*t188+t109.*t191-t2.*t6.*t155)+dphi2.*(t155.*t223+t157.*t227-t188.*t232+t191.*t231-t193.*t236-t194.*t235);
et5 = dth1.*(t155.*t228+t156.*t227-t174.*t236-t175.*t235-t188.*t229+t191.*t230)+dx.*(t12.*t155-t4.*t6.*t191+t6.*t10.*t188)-t5.*t188.*windspeed+t11.*t191.*windspeed;
aoa_tail_5 = th2-atan((et4+et5)./(et1+et2+et3));
